simulink model "Arneodo"  (R2014b)
settings: Solver=ode45  StartTime=0.0  StopTime=10.0  RelTol=1e-3
values from neighbouring files (symbols this model uses):
  a = 0.95    [Run_Aizawa.m]    (also in Run_Arneodo.m = -5.5; Run_Chen.m = 33; Run_Chua.m = 15.6; Run_Chua_4D.m = 0.03)
  b = 0.7    [Run_Aizawa.m]    (also in Run_Arneodo.m = 3.5; Run_Chen.m = 3; Run_Chua.m = 28; Run_Duffing.m = 100)
  c = -1    [Run_Arneodo.m]    (also in Run_Chen.m = 25; Run_Chua_4D.m = -1.2; Run_Dadras.m = 2; Run_HindmarshRose.m = 1)
undefined symbols (not defined in the file or in its folder): param
settings Model: Creator=Arek  LastModifiedBy=Arek

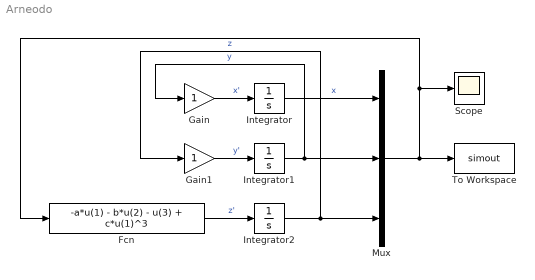
== system Arneodo ==
  Fcn : Fcn  Expr=-a*u(1) - b*u(2) - u(3) + c*u(1)^3
  Gain : Gain
  Gain1 : Gain
  Integrator : Integrator  InitialCondition=param.ic(1)
  Integrator1 : Integrator  InitialCondition=param.ic(2)
  Integrator2 : Integrator  InitialCondition=param.ic(3)
  Mux : Mux  Inputs=3
  Scope : Scope
      settings: ShowLegends=on
  To Workspace : ToWorkspace  VariableName=simout  SaveFormat=Timeseries  SampleTime=-1
  wires:
  Gain/1 -> Integrator/1  "x'"
  Integrator/1 -> Mux/1  "x"
  Integrator1/1 -> Mux/2, Gain/1  "y"
  Fcn/1 -> Integrator2/1  "z'"
  Integrator2/1 -> Mux/3, Gain1/1  "z"
  Gain1/1 -> Integrator1/1  "y'"
  Mux/1 -> Scope/1, Fcn/1, To Workspace/1
